simulink model "MBSimulation"  (R2017a)
settings: Solver=VariableStepAuto  StartTime=0.0  StopTime=10  RelTol=1e-3
settings Model: Creator=tnorris  LastModifiedBy=tnorris
settings SolverCC: MaxConsecutiveMinStep=100

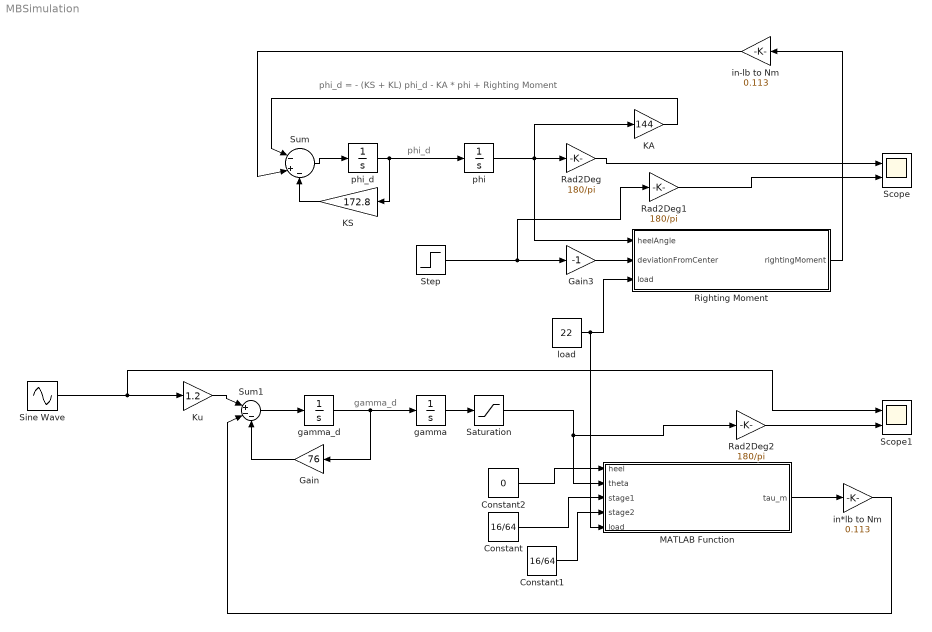
== system MBSimulation ==
  note: phi_d = - (KS + KL) phi_d - KA * phi + Righting Moment
  note: gamma_d
  note: phi_d
  Constant : Constant  Value=16/64
  Constant1 : Constant  Value=16/64
  Constant2 : Constant  Value=0
  Gain : Gain  Gain=76
  Gain3 : Gain  Gain=-1
  KA : Gain  Gain=144
  "KS " : Gain  Gain=172.8
  Ku : Gain  Gain=1.2
  MATLAB Function : MATLAB Function  TreatAsAtomicUnit=on
  "Rad2Deg " : Gain  Gain=180/pi
  Rad2Deg1 : Gain  Gain=180/pi
  Rad2Deg2 : Gain  Gain=180/pi
  Righting Moment : MATLAB Function  TreatAsAtomicUnit=on
  Saturation : Saturate  UpperLimit=pi/4  LowerLimit=-pi/4
  Scope : Scope  NumInputPorts=2
  Scope1 : Scope  NumInputPorts=2
  Sine Wave : Sin  Amplitude=12  SampleTime=0
  Step : Step  After=pi/4  SampleTime=0
  Sum : Sum  Inputs=|-+-
  Sum1 : Sum  Inputs=|+--
  gamma : Integrator  InitialCondition=.0
  gamma_d : Integrator
  in*lb to Nm : Gain  Gain=0.113
  in-lb to Nm : Gain  Gain=0.113
  load : Constant  Value=22
  phi : Integrator
  phi_d : Integrator
  wires:
  gamma_d/1 -> Gain/1, gamma/1
  Sum/1 -> phi_d/1
  Sum1/1 -> gamma_d/1
  Ku/1 -> Sum1/1
  KA/1 -> Sum/1
  gamma/1 -> Saturation/1
  load/1 -> MATLAB Function/5(load), Righting Moment/3(load)
  Constant/1 -> MATLAB Function/3(stage1)
  Constant1/1 -> MATLAB Function/4(stage2)
  Gain/1 -> Sum1/3
  phi/1 -> "Rad2Deg "/1, Righting Moment/1(heelAngle), KA/1
  phi_d/1 -> "KS "/1, phi/1
  MATLAB Function/1(tau_m) -> in*lb to Nm/1
  in*lb to Nm/1 -> Sum1/2
  "Rad2Deg "/1 -> Scope/1
  Rad2Deg1/1 -> Scope/2
  Step/1 -> Gain3/1, Rad2Deg1/1
  Righting Moment/1(rightingMoment) -> in-lb to Nm/1
  in-lb to Nm/1 -> Sum/2
  "KS "/1 -> Sum/3
  Gain3/1 -> Righting Moment/2(deviationFromCenter)
  Constant2/1 -> MATLAB Function/1(heel)
  Saturation/1 -> Rad2Deg2/1, MATLAB Function/2(theta)
  Sine Wave/1 -> Scope1/1, Ku/1
  Rad2Deg2/1 -> Scope1/2

== matlab function MBSimulation/MATLAB Function ==
  data: heel input; tau_m output; theta input; stage1 input; stage2 input; load input
function tau_m   = calcMBTorque( heel, theta, stage1, stage2,  load)
  shaftElev = 28.6 * pi / 180.0;
  grav = [0; 0; -1];
  % Start in inertial (X=North, Y=West, Z=Up)
  % Transform onto boat (X=Forward, Y=Port, Z=Up along mast)
  R_world_boat = [1 0 0;
                  0 cos(heel) sin(heel);
                  0 -sin(heel) cos(heel)];
  grav_boat = R_world_boat * grav;
  % Tilt to shaft (X=Forward/Up along tilt, Y=Port, Z=Up/Tilted back)
  R_boat_shaft = [cos(shaftElev) 0 sin(shaftElev);
                  0              1 0;
                  -sin(shaftElev) 0 cos(shaftElev)];
  grav_shaft = R_boat_shaft * grav_boat;
  % Rotate to position of MB (X=straight out on arm, Y=Orthogonal to X
  %   in plane of arm sweep, Z=along shaft)
  R_shaft_mb = [cos(theta) sin(theta) 0;
                -sin(theta) cos(theta) 0;
                0 0 1];
  grav_mb = R_shaft_mb * grav_shaft;
  % The gravity along the Y-axis will produce the torque
  armLen = 25.25;
  tau = grav_mb(2) * armLen;

  effectiveLoad = load*tau;

  tau_m = effectiveLoad*stage1*stage2/0.9/0.9;

end

== matlab function MBSimulation/Righting Moment ==
  data: heelAngle input; rightingMoment output; deviationFromCenter input; load input
function rightingMoment   = calcMBRightingMoment(heelAngle, deviationFromCenter, load )
%UNTITLED Summary of this function goes here
%   Detailed explanation goes here
MBShaftElevation = deg2rad(28.6); % deg
verticalShaftOffset = 7.21; % in

tf_BoatCenterline_Heeled = calcTransform(0, heelAngle,0, pi/2);
tf_Heeled_ShaftBase = calcTransform(verticalShaftOffset, 0, 0, MBShaftElevation);
tf_ShaftBase_ArmCS = calcTransform(0, deviationFromCenter, 0, 0);

tf_WCS_ArmCS = tf_BoatCenterline_Heeled*tf_Heeled_ShaftBase*tf_ShaftBase_ArmCS;

armInWCS = tf_WCS_ArmCS*[0; 25.25; -7.9; 1];

rightingMoment = armInWCS(1)*load;

end
